simulink model "PMSM_DBPC"  (R2024b)
settings: Solver=FixedStepDiscrete  StartTime=0.0  StopTime=0.8  FixedStep=1e-6  RelTol=1e-3
libraries: spsMosfetLib x12, spsDiodeLib x6, spsCurrentMeasurementLib x6, spsVoltageMeasurementLib x5, spsSeriesRLCBranchLib x4, spsDCVoltageSourceLib x3, simulink x2, spsOnDelayLib x1, slpidlib x1, spsPermanentMagnetSynchronousMachineLib x1, spspowerguiLib x1
settings Model: Creator=23230  LastModifiedBy=23230

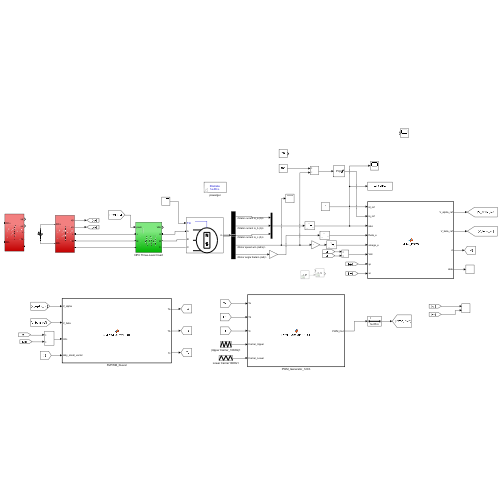
[thumbnail: Simulink's stored preview of the top-level diagram]
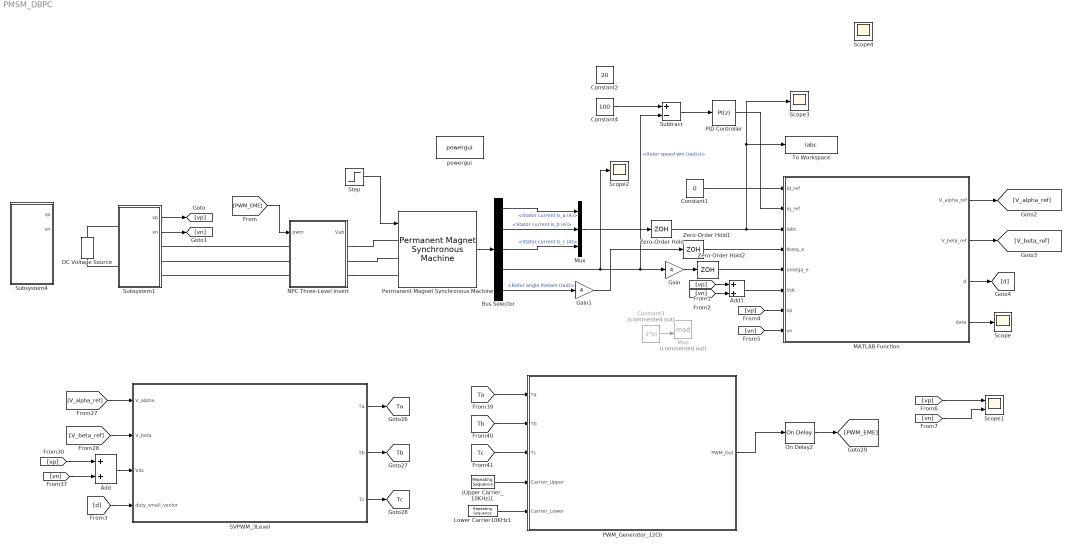
== system PMSM_DBPC ==
  (Upper Carrier_10KHz)1 : simulink/Sources/Repeating Sequence  rep_seq_t=[0, 5e-5, 1e-4]  rep_seq_y=[0.5, 1, 0.5]
  Add : Sum
  Add1 : Sum
  Bus Selector : BusSelector  OutputSignals=Stator current is_a (A),Stator current is_b (A),Stator current is_c (A),Rotor speed wm (rad/s),Rotor angle thetam (rad)
  Constant1 : Constant  Value=0
  Constant2 : Constant  Value=20
  Constant3 : Constant  Commented=on  Value=2*pi
  Constant4 : Constant  Value=100
  DC Voltage Source : spsDCVoltageSourceLib/DC Voltage Source  Amplitude=600  Measurements=None
  Gain : Gain  Gain=4
  Gain1 : Gain  Gain=4
  Lower Carrier10KHz1 : simulink/Sources/Repeating Sequence  rep_seq_t=[0, 5e-5, 1e-4]  rep_seq_y=[0, 0.5, 0]
  MATLAB Function : MATLAB Function  TreatAsAtomicUnit=on
  Mod : Math  Commented=on  Operator=mod
  Mux : Mux  Inputs=3
  NPC Three-Level Invert : Subsystem
  On Delay2 : spsOnDelayLib/On Delay  DelayType=On delay  delay=1e-6  ic=0  Ts=0
  PID Controller : slpidlib/PID Controller  Controller=PI  Form=Parallel  TimeDomain=Discrete-time  UseExternalTs=off  SampleTime=-1  IntegratorMethod=Forward Euler  FilterMethod=Forward Euler  ControllerParametersSource=internal  P=5  I=50  UseKiTs=off  D=0  UseExternalDerivativeSource=off  N=100  UseFilter=on  TunerSelectOption=Transfer Function Based (PID Tuner App)  InitialConditionSource=internal  InitialConditionForIntegrator=0  InitialConditionForFilter=0  DifferentiatorICPrevScaledInput=0  ExternalReset=none  TrackingMode=off  Kt=1  LimitOutput=on  SatLimitsSource=internal  UpperSaturationLimit=40  LowerSaturationLimit=-40  LinearizeAsGain=on  AntiWindupMode=none  Kb=1  LimitIntegrator=off  UpperIntegratorSaturationLimit=inf  LowerIntegratorSaturationLimit=-inf  POutMin=[]  POutMax=[]  IOutMin=[]  IOutMax=[]  DOutMin=[]  DOutMax=[]  NOutMin=[]  NOutMax=[]  SumOutMin=[]  SumOutMax=[]  SaturationOutMin=[]  SaturationOutMax=[]  PParamMin=[]  PParamMax=[]  IParamMin=[]  IParamMax=[]  DParamMin=[]  DParamMax=[]  NParamMin=[]  NParamMax=[]  KbParamMin=[]  KbParamMax=[]  KtParamMin=[]  KtParamMax=[]  KbOutMin=[]  KbOutMax=[]  KtOutMin=[]  KtOutMax=[]  IntegratorOutMin=[]  IntegratorOutMax=[]  FilterOutMin=[]  FilterOutMax=[]  SumI1OutMin=[]  SumI1OutMax=[]  SumI2OutMin=[]  SumI2OutMax=[]  SumI3OutMin=[]  SumI3OutMax=[]  SumI4OutMin=[]  SumI4OutMax=[]  SumDOutMin=[]  SumDOutMax=[]  DifferentiatorOutMin=[]  DifferentiatorOutMax=[]  FilterDiffOutCoefMin=[]  FilterDiffOutCoefMax=[]  ReciprocalOutMin=[]  ReciprocalOutMax=[]  SumDenOutMin=[]  SumDenOutMax=[]  SumNumOutMin=[]  SumNumOutMax=[]  DivideOutMin=[]  DivideOutMax=[]  UdiffTsProdOutMin=[]  UdiffTsProdOutMax=[]  NTsProdOutMin=[]  NTsProdOutMax=[]  UintegralTsProdOutMin=[]  UintegralTsProdOutMax=[]  UngainTsProdOutMin=[]  UngainTsProdOutMax=[]  ClampingZeroOutDataTypeStr=Inherit: Inherit via back propagation  ClampingZeroOutMin=[]  ClampingZeroOutMax=[]  FilterDenConstantOutDataTypeStr=Inherit: Inherit via back propagation  FilterDenConstantOutMin=[]  FilterDenConstantOutMax=[]  PCopyOutDataTypeStr=Inherit: Inherit via back propagation  PCopyOutMin=[]  PCopyOutMax=[]  NCopyOutDataTypeStr=Inherit: Inherit via back propagation  NCopyOutMin=[]  NCopyOutMax=[]  IntegratorContinuousStateAttributes=''  IntegratorStateMustResolveToSignalObject=off  IntegratorRTWStateStorageClass=Auto  FilterContinuousStateAttributes=''  FilterStateMustResolveToSignalObject=off  FilterRTWStateStorageClass=Auto  ParallelPVariant=InternalParameters  IdealPVariant=Disabled  IVariant=InternalParameters  DVariant=Disabled  IntegratorVariant=Discrete  SatVariant=Enabled  AWVariant=Passthrough  PCopyVariant=Disabled  TRVariant=Disabled  FdbkBlocksVariant=Forward  IdealPFdbkVariant=Disabled  SatFdbkVariant=Disabled  DerivativeFilterVariant=Disabled  NVariant=Disabled  NCopyVariant=Disabled_SignalSpec  FilterICVariant=Disabled  IntegratorICVariant=InternalICs  ExternalResetVariant=Disabled  TRSumVariant=Passthrough  SumFdbkVariant=Disabled  SumVariant=Sum_PI  TsampFilterVariant=InternalTs  TsampNgainVariant=Passthrough  TsampIntegralVariant=Disabled_SignalSpec  ExternalSaturationOutDataTypeStr=Inherit: Same as second input  DerivativeSourceVariant=Disabled  PreIntVariant=InternalPreInt
  PWM_Generator_12Ch : MATLAB Function  TreatAsAtomicUnit=on
  Permanent Magnet Synchronous Machine : spsPermanentMagnetSynchronousMachineLib/Permanent Magnet Synchronous Machine  NbPhases=3  FluxDistribution=Sinusoidal  RotorType=Round  MechanicalLoad=Torque Tm  PresetModel=No  ShowDetailedParameters=on  MeasurementBus=off  Resistance=0.015  Inductance=8.5e-3  dqInductances=[8.5e-3,8.5e-3]  La=0.00025  MachineConstant=Flux linkage established by magnets (V.s)  Flux=0.08  VoltageCst=58.0416  TorqueCst=0.48  Flat=120  Mechanical=[0.0027 0.0004924 4 0]  PolePairs=4  InitialConditions=[0,0, 0,0]  InitialConditions5ph=[0 0 0 0 0 0]  RefAngle=Aligned with phase A axis (original Park)  IterativeDiscreteModel=Trapezoidal non iterative  TsBlock=-1  TsPowergui=0
  SVPWM_3Level : MATLAB Function  TreatAsAtomicUnit=on
  Scope{,2..4} (4 alike) : Scope
  Scope1 : Scope  NumInputPorts=2
  Step : Step  Time=0.15  Before=5  After=15  SampleTime=0
  Subsystem1 : Subsystem
  Subsystem4 : Subsystem
  Subtract : Sum  Inputs=+-
  To Workspace : ToWorkspace  VariableName=iabc  SaveFormat=Timeseries  SampleTime=-1
  Zero-Order Hold : ZeroOrderHold  SampleTime=1e-4
  Zero-Order Hold1 : ZeroOrderHold  SampleTime=1e-4
  Zero-Order Hold2 : ZeroOrderHold  SampleTime=1e-4
  powergui : spspowerguiLib/powergui  Priority=1  SimulationMode=Discrete  SampleTime=1e-6  frequency=60  Iterations=50  frequencyindice=0  Pbase=100e6  ErrMax=1e-4  UnitsV=kV  UnitsW=MW  buscounter=0  FunctionMessages=off  echomessages=off  EnableUseOfTLC=off  CurrentSourceSwitches=off  DisableSnubberDevices=off  DisableRonSwitches=off  DisableVfSwitches=off  DisplayEquations=off  AutomaticDiscreteSolvers=off  SolverType=Tustin/Backward Euler (TBE)  Interpol=off  ExternalGateDelay=off  methode=off  Ts=100  x0status=blocks  SPID=on  SwTol=0  HookPort=off  NonlinearTolerance=1e-4  nMaxIteration=100  ContinueOnMaxIteration=off  RestoreLinks=warning  ResistiveCurrentMeasurement=off  Frange=[0:2:500]  Ylog=off  Xlog=on  ShowGrid=off  save=off  variable=ZData  structure=0  ZoomFFT=off  StartTime=0.0  cycles=1  DisplayStyle=1  fundamental=60  FreqAxis=off  MaxFrequency=1000  frequencyindicesteady=1  RmsSteady=1  display=off
  tag scope: Ta=global, Tb=global, Tc=global
  wires:
  Constant1/1 -> MATLAB Function/1(id_ref)
  [vp] -> Add/1
  [vn] -> Add/2
  [V_beta_ref] -> SVPWM_3Level/2(V_beta)
  [V_alpha_ref] -> SVPWM_3Level/1(V_alpha)
  SVPWM_3Level/1(Ta) -> [Ta]
  SVPWM_3Level/3(Tc) -> [Tc]
  SVPWM_3Level/2(Tb) -> [Tb]
  Add/1 -> SVPWM_3Level/3(Vdc)
  [Tc] -> PWM_Generator_12Ch/3(Tc)
  Lower Carrier10KHz1/1 -> PWM_Generator_12Ch/5(Carrier_Lower)
  On Delay2/1 -> [PWM_EME]
  (Upper Carrier_10KHz)1/1 -> PWM_Generator_12Ch/4(Carrier_Upper)
  PWM_Generator_12Ch/1(PWM_Out) -> On Delay2/1
  [Ta] -> PWM_Generator_12Ch/1(Ta)
  [Tb] -> PWM_Generator_12Ch/2(Tb)
  [PWM_EME] -> NPC Three-Level Invert/1(pwm)
  Permanent Magnet Synchronous Machine/1 -> Bus Selector/1
  Bus Selector/1 -> Mux/1  "<Stator current is_a (A)>"
  Bus Selector/2 -> Mux/2  "<Stator current is_b (A)>"
  Bus Selector/3 -> Mux/3  "<Stator current is_c (A)>"
  Mux/1 -> Zero-Order Hold/1
  Bus Selector/4 -> Scope2/1, Subtract/2, Gain/1  "<Rotor speed wm (rad/s)>"
  Gain/1 -> Zero-Order Hold2/1
  Bus Selector/5 -> Gain1/1  "<Rotor angle thetam (rad)>"
  Constant3/1 -> Mod/2
  [d] -> SVPWM_3Level/4(duty_small_vector)
  MATLAB Function/1(V_alpha_ref) -> [V_alpha_ref]
  MATLAB Function/2(V_beta_ref) -> [V_beta_ref]
  MATLAB Function/4(data) -> Scope/1
  [vn] -> Add1/2
  [vp] -> Add1/1
  Add1/1 -> MATLAB Function/6(Vdc)
  Zero-Order Hold/1 -> To Workspace/1, Scope3/1, MATLAB Function/3(iabc)
  Zero-Order Hold1/1 -> MATLAB Function/4(theta_e)
  Zero-Order Hold2/1 -> MATLAB Function/5(omega_e)
  Gain1/1 -> Zero-Order Hold1/1
  Subsystem1/1(vp) -> [vp]
  Subsystem1/2(vn) -> [vn]
  MATLAB Function/3(d) -> [d]
  [vp] -> MATLAB Function/7(vp)
  [vn] -> MATLAB Function/8(vn)
  [vp] -> Scope1/1
  [vn] -> Scope1/2
  Constant4/1 -> Subtract/1
  Subtract/1 -> PID Controller/1
  PID Controller/1 -> MATLAB Function/2(iq_ref)
  Step/1 -> Permanent Magnet Synchronous Machine/1
  connections:
  NPC Three-Level Invert/RConn1 -- Permanent Magnet Synchronous Machine/LConn1
  NPC Three-Level Invert/RConn2 -- Permanent Magnet Synchronous Machine/LConn2
  NPC Three-Level Invert/RConn3 -- Permanent Magnet Synchronous Machine/LConn3
  NPC Three-Level Invert/LConn1 -- Subsystem1/RConn1
  NPC Three-Level Invert/LConn2 -- Subsystem1/RConn2
  NPC Three-Level Invert/LConn3 -- Subsystem1/RConn3
  DC Voltage Source/RConn1 -- Subsystem1/LConn1
  DC Voltage Source/LConn1 -- Subsystem1/LConn2

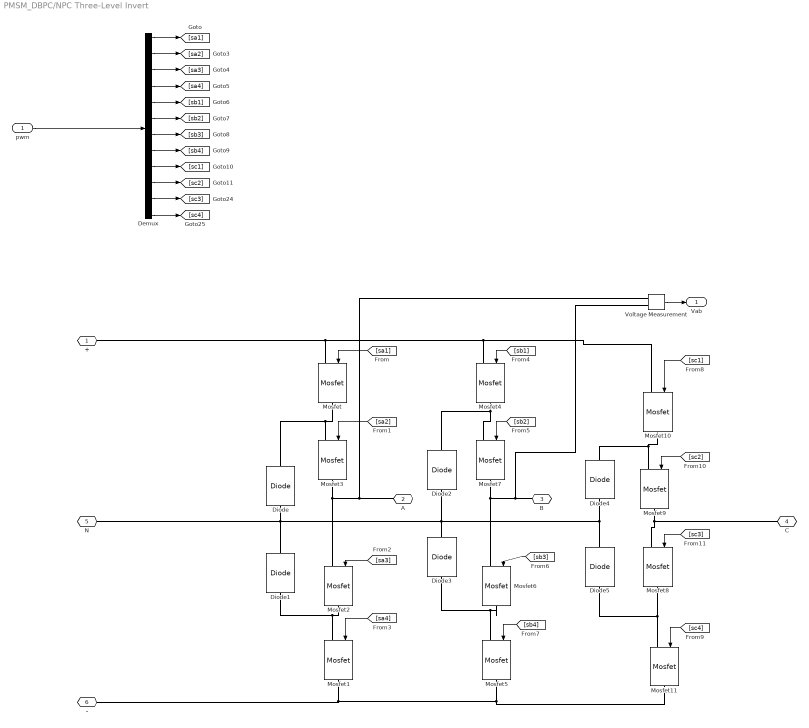
== system PMSM_DBPC/NPC Three-Level Invert ==
  pwm : Inport
  Demux : Demux  Outputs=12
  Diode{,1..5} (6 alike) : spsDiodeLib/Diode  Ron=0.001  Lon=0  Vf=0.8  IC=0  UseSnubber=0  Rs=500  Cs=250e-9  Measurements=off
  Mosfet{,1..11} (12 alike) : spsMosfetLib/Mosfet  Ron=0.1  Lon=0  Rd=0.01  Vfd=0  IC=0  Rs=1e5  Cs=inf  Measurements=off
  Voltage Measurement : spsVoltageMeasurementLib/Voltage Measurement  PhasorSimulation=off  OutputType=Complex  PSBequivalent=0
  + : PMIOPort  Side=Left
  A : PMIOPort  Port=2  Side=Right
  B : PMIOPort  Port=3  Side=Right
  C : PMIOPort  Port=4  Side=Right
  N : PMIOPort  Port=5  Side=Left
  - : PMIOPort  Port=6  Side=Left
  Vab : Outport
  wires:
  [sb2] -> Mosfet7/1
  [sc3] -> Mosfet8/1
  [sa4] -> Mosfet1/1
  Demux/2 -> [sa2]
  Demux/10 -> [sc2]
  Demux/7 -> [sb3]
  Demux/4 -> [sa4]
  Demux/11 -> [sc3]
  [sb3] -> Mosfet6/1
  [sc1] -> Mosfet10/1
  [sc4] -> Mosfet11/1
  Demux/9 -> [sc1]
  [sa1] -> Mosfet/1
  Demux/1 -> [sa1]
  Demux/12 -> [sc4]
  [sa3] -> Mosfet2/1
  [sc2] -> Mosfet9/1
  [sb1] -> Mosfet4/1
  Demux/5 -> [sb1]
  [sb4] -> Mosfet5/1
  [sa2] -> Mosfet3/1
  Demux/6 -> [sb2]
  Demux/3 -> [sa3]
  Demux/8 -> [sb4]
  Voltage Measurement/1 -> Vab/1
  pwm/1 -> Demux/1
  connections:
  Mosfet/RConn1 -- Diode/RConn1 -- Mosfet3/LConn1
  Mosfet9/RConn1 -- C/RConn1 -- Mosfet8/LConn1
  Mosfet9/LConn1 -- Diode4/RConn1 -- Mosfet10/RConn1
  Diode3/RConn1 -- Diode5/RConn1 -- Diode4/LConn1 -- Diode2/LConn1 -- Diode1/RConn1 -- N/RConn1 -- Diode/LConn1
  Mosfet/LConn1 -- +/RConn1 -- Mosfet10/LConn1 -- Mosfet4/LConn1
  Mosfet8/RConn1 -- Diode5/LConn1 -- Mosfet11/LConn1
  Mosfet2/RConn1 -- Diode1/LConn1 -- Mosfet1/LConn1
  Mosfet1/RConn1 -- -/RConn1 -- Mosfet11/RConn1 -- Mosfet5/RConn1
  Mosfet3/RConn1 -- Mosfet2/LConn1 -- Voltage Measurement/LConn1 -- A/RConn1
  Mosfet6/RConn1 -- Diode3/LConn1 -- Mosfet5/LConn1
  Mosfet7/RConn1 -- Mosfet6/LConn1 -- Voltage Measurement/LConn2 -- B/RConn1
  Mosfet4/RConn1 -- Diode2/RConn1 -- Mosfet7/LConn1

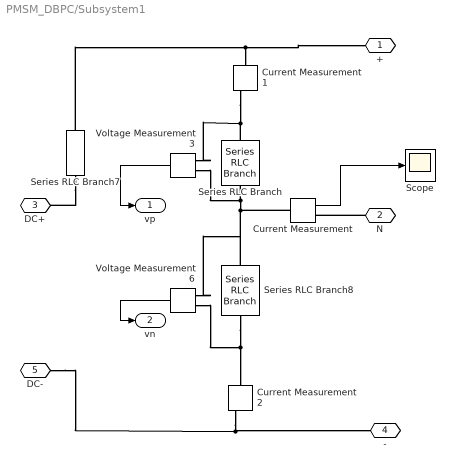
== system PMSM_DBPC/Subsystem1 ==
  Current Measurement : spsCurrentMeasurementLib/Current Measurement  PhasorSimulation=off  OutputType=Complex  PSBequivalent=0
  Current Measurement1 : spsCurrentMeasurementLib/Current Measurement  PhasorSimulation=off  OutputType=Complex  PSBequivalent=0
  Current Measurement2 : spsCurrentMeasurementLib/Current Measurement  PhasorSimulation=off  OutputType=Complex  PSBequivalent=0
  Scope : Scope
  Series RLC Branch : spsSeriesRLCBranchLib/Series RLC Branch  LConnTagsString=__new0  RConnTagsString=__new0  BranchType=C  Resistance=1  Inductance=1e-3  SetiL0=off  InitialCurrent=0  Capacitance=470e-6  Setx0=on  InitialVoltage=300  Measurements=Branch current
  Series RLC Branch7 : spsSeriesRLCBranchLib/Series RLC Branch  LConnTagsString=__new0  RConnTagsString=__new0  BranchType=R  Resistance=0.0001  Inductance=1e-3  SetiL0=off  InitialCurrent=0  Capacitance=1e-6  Setx0=off  InitialVoltage=0  Measurements=None
  Series RLC Branch8 : spsSeriesRLCBranchLib/Series RLC Branch  LConnTagsString=__new0  RConnTagsString=__new0  BranchType=C  Resistance=1  Inductance=1e-3  SetiL0=off  InitialCurrent=0  Capacitance=470e-6  Setx0=on  InitialVoltage=300  Measurements=Branch current
  Voltage Measurement3 : spsVoltageMeasurementLib/Voltage Measurement  PhasorSimulation=off  OutputType=Complex  PSBequivalent=0
  Voltage Measurement6 : spsVoltageMeasurementLib/Voltage Measurement  PhasorSimulation=off  OutputType=Complex  PSBequivalent=0
  + : PMIOPort  Side=Right
  N : PMIOPort  Port=2  Side=Right
  DC+ : PMIOPort  Port=3  Side=Left
  - : PMIOPort  Port=4  Side=Right
  DC- : PMIOPort  Port=5  Side=Left
  vp : Outport
  vn : Outport  Port=2
  wires:
  Voltage Measurement3/1 -> vp/1
  Voltage Measurement6/1 -> vn/1
  Current Measurement/1 -> Scope/1
  connections:
  Series RLC Branch7/RConn1 -- Current Measurement1/LConn1 -- +/RConn1
  Series RLC Branch/RConn1 -- Voltage Measurement3/LConn2 -- Series RLC Branch8/LConn1 -- Voltage Measurement6/LConn1 -- Current Measurement/LConn1
  Series RLC Branch8/RConn1 -- Current Measurement2/LConn1 -- Voltage Measurement6/LConn2
  Series RLC Branch7/LConn1 -- DC+/RConn1
  N/RConn1 -- Current Measurement/RConn1
  Current Measurement1/RConn1 -- Voltage Measurement3/LConn1 -- Series RLC Branch/LConn1
  Current Measurement2/RConn1 -- -/RConn1 -- DC-/RConn1

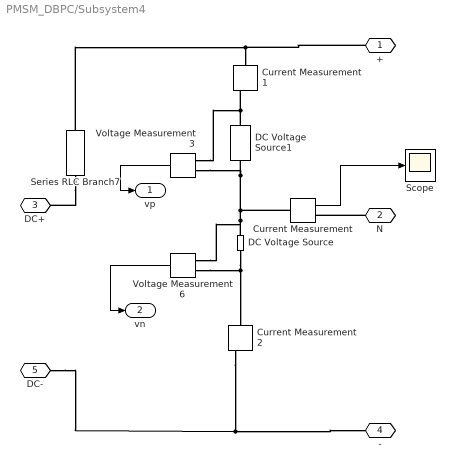
== system PMSM_DBPC/Subsystem4 ==
  Current Measurement : spsCurrentMeasurementLib/Current Measurement  PhasorSimulation=off  OutputType=Complex  PSBequivalent=0
  Current Measurement1 : spsCurrentMeasurementLib/Current Measurement  PhasorSimulation=off  OutputType=Complex  PSBequivalent=0
  Current Measurement2 : spsCurrentMeasurementLib/Current Measurement  PhasorSimulation=off  OutputType=Complex  PSBequivalent=0
  DC Voltage Source : spsDCVoltageSourceLib/DC Voltage Source  Amplitude=300  Measurements=None
  DC Voltage Source1 : spsDCVoltageSourceLib/DC Voltage Source  Amplitude=300  Measurements=None
  Scope : Scope
  Series RLC Branch7 : spsSeriesRLCBranchLib/Series RLC Branch  LConnTagsString=__new0  RConnTagsString=__new0  BranchType=R  Resistance=0.0001  Inductance=1e-3  SetiL0=off  InitialCurrent=0  Capacitance=1e-6  Setx0=off  InitialVoltage=0  Measurements=None
  Voltage Measurement3 : spsVoltageMeasurementLib/Voltage Measurement  PhasorSimulation=off  OutputType=Complex  PSBequivalent=0
  Voltage Measurement6 : spsVoltageMeasurementLib/Voltage Measurement  PhasorSimulation=off  OutputType=Complex  PSBequivalent=0
  + : PMIOPort  Side=Right
  N : PMIOPort  Port=2  Side=Right
  DC+ : PMIOPort  Port=3  Side=Left
  - : PMIOPort  Port=4  Side=Right
  DC- : PMIOPort  Port=5  Side=Left
  vp : Outport
  vn : Outport  Port=2
  wires:
  Voltage Measurement3/1 -> vp/1
  Voltage Measurement6/1 -> vn/1
  Current Measurement/1 -> Scope/1
  connections:
  Series RLC Branch7/RConn1 -- +/RConn1 -- Current Measurement1/LConn1
  DC Voltage Source/LConn1 -- Current Measurement2/LConn1 -- Voltage Measurement6/LConn2
  Series RLC Branch7/LConn1 -- DC+/RConn1
  N/RConn1 -- Current Measurement/RConn1
  Current Measurement2/RConn1 -- -/RConn1 -- DC-/RConn1
  DC Voltage Source1/RConn1 -- Voltage Measurement3/LConn1 -- Current Measurement1/RConn1
  DC Voltage Source/RConn1 -- Voltage Measurement3/LConn2 -- DC Voltage Source1/LConn1 -- Current Measurement/LConn1 -- Voltage Measurement6/LConn1

== matlab function PMSM_DBPC/MATLAB Function ==
  data: id_ref input; V_alpha_ref output; iq_ref input; iabc input; theta_e input; omega_e input; Vdc input; V_beta_ref output; d output; data output; vp input; vn input
function [V_alpha_ref, V_beta_ref, d, data] = Motor_DBPC(id_ref, iq_ref, iabc, theta_e, omega_e, Vdc, vp, vn)
    % ==========================================================
    % 永磁同步电机多目标解析无差拍预测控制 (MO-DBPC) 
    % 包含：1. 前馈+抗饱和条件积分复合控制 (彻底消除稳态静差且防爆炸)
    %       2. 基于电荷预测的多目标中点电位平衡控制
    % ==========================================================
    
    % --- 0. 物理参数定义 ---
    Ts = 1e-4;         % 采样周期 (s)
    Rs = 0.015;        % 定子电阻 (Ohm)
    Ld = 0.00025;      % d轴电感 (H)
    Lq = 0.00025;      % q轴电感 (H)
    psi_f = 0.08;      % 永磁体磁链 (Wb)
    C_cap = 470e-6;    % 直流侧单电容容量 (F)
    
    % --- 1. 坐标变换 (abc -> alpha/beta -> d/q) ---
    T_clark = (2/3) * [1, -0.5, -0.5; 0, sqrt(3)/2, -sqrt(3)/2];
    i_ab = T_clark * iabc;
    i_alpha = i_ab(1);
    i_beta  = i_ab(2);
    
    id =  i_alpha * cos(theta_e) + i_beta * sin(theta_e);
    iq = -i_alpha * sin(theta_e) + i_beta * cos(theta_e);
    
    % --- 2. 电流追踪：前馈无差拍 + 条件积分补偿 (消除静差) ---
    % 声明持久化变量，作为离散积分器的记忆单元
    persistent ud_int uq_int;
    if isempty(ud_int)
        ud_int = 0;
        uq_int = 0;
    end
    
    % 积分控制器参数 (针对 1e-4 极小步长优化)
    Ki = 0.005;        % 极小积分增益，保证稳态微调的平滑性
    Int_Limit = 15;    % 积分抗饱和限幅值 (V)，防止超调翻车
    
    % 计算当前拍的电流静差
    err_d = id_ref - id;
    err_q = iq_ref - iq;
    
    % 【核心修复】：条件积分 (Conditional Integration)
    % 仅在误差小于 5A 时开启积分，完美避开启动和突加负载瞬间的 Windup 爆炸
    if abs(err_d) < 5
        ud_int = ud_int + Ki * err_d;
    end
    
    if abs(err_q) < 5
        uq_int = uq_int + Ki * err_q;
    end
    
    % 抗饱和限幅 (最后的一道安全锁)
    ud_int = max(-Int_Limit, min(Int_Limit, ud_int));
    uq_int = max(-Int_Limit, min(Int_Limit, uq_int));
    
    % 复合控制电压求解：DBPC物理前馈(定大局) + 误差积分补偿(修毫厘)
    ud_ref = Rs * id + (Ld / Ts) * (id_ref - id) - omega_e * Lq * iq + ud_int;
    uq_ref = Rs * iq + (Lq / Ts) * (iq_ref - iq) + omega_e * Ld * id + omega_e * psi_f + uq_int;
    
    % --- 3. 逆坐标变换 (d/q -> alpha/beta) ---
    V_alpha_ref = ud_ref * cos(theta_e) - uq_ref * sin(theta_e);
    V_beta_ref  = ud_ref * sin(theta_e) + uq_ref * cos(theta_e);
    
    % --- 4. 【核心创新】：改进多目标解析无差拍中点控制 ---
    delta_v = vp - vn; % 当前中点电压偏差
    
    % 扇区判断 (根据参考电压矢量定位)
    theta_v = atan2(V_beta_ref, V_alpha_ref);
    if theta_v < 0, theta_v = theta_v + 2*pi; end
    Sector = floor(theta_v / (pi/3)) + 1;
    if Sector > 6, Sector = 6; end
    
    % 根据扇区提取可能流过中点的相电流
    switch Sector
        case 1, i_p = iabc(1);  i_n = -iabc(1); 
        case 2, i_p = -iabc(3); i_n = iabc(3);
        case 3, i_p = iabc(2);  i_n = -iabc(2);
        case 4, i_p = -iabc(1); i_n = iabc(1);
        case 5, i_p = iabc(3);  i_n = -iabc(3);
        case 6, i_p = -iabc(2); i_n = iabc(2);
        otherwise, i_p = 0; i_n = 0;
    end
    
    % 解析求解最优分配因子 d
    denominator = i_p - i_n;
    if abs(denominator) < 0.1
        % 如果中点电流激励过小，为防止除以0的奇异点，直接均分
        d = 0.5; 
    else
        % 多目标解析解：兼顾电压平衡 (lambda_v) 与 电流平滑 (lambda_cmv)
        lambda_v   = 1.0;  
        lambda_cmv = 0.005; % THD与电压波动的最优折中权重
        
        % 代价函数求导后的代数解析解计算
        A = (Ts / C_cap) * denominator;
        V_req = delta_v - (Ts / C_cap) * i_n;
        d = (lambda_v * A * V_req + 0.5 * lambda_cmv) / (lambda_v * A^2 + lambda_cmv);
    end
    
    % 占空比物理约束
    d = max(0.0, min(1.0, d));
    
    % 导出数据供示波器观察
    data = [id; iq; id_ref; iq_ref; delta_v; d]; 
end

== matlab function PMSM_DBPC/SVPWM_3Level ==
  data: V_alpha input; Ta output; V_beta input; Vdc input; duty_small_vector input; Tb output; Tc output
function [Ta, Tb, Tc] = SVPWM_3Level_Full(V_alpha, V_beta, Vdc, duty_small_vector)
    % ==========================================================
    % 三电平 NPC 逆变器空间矢量调制 (全扇区映射版)
    % 集成 DBPC 冗余小矢量非对称分配 (协同控制电容电压与零序电流)
    % 【最终完美版】：已修复 atan2 下半圆负角度导致的停工 Bug
    % ==========================================================
    
    % --- 1. 参考电压极坐标转换 ---
    V_ref = sqrt(V_alpha^2 + V_beta^2);
    theta = atan2(V_beta, V_alpha);
    
    % ==========================================================
    % 【救命补丁：防止下半平面角度变负数，导致逆变器罢工！】
    % ==========================================================
    if theta < 0
        theta = theta + 2*pi;
    end
    
    % 计算调制比
    m = sqrt(3) * V_ref / Vdc; 
    
    % --- 2. 扇区判断 (Sector 1 ~ 6) ---
    Sector = floor(theta / (pi/3)) + 1;
    if Sector > 6
        Sector = 6; % 安全保护
    end
    
    % --- 3. 核心：扇区对称映射 ---
    if mod(Sector, 2) == 0
        theta_rel = pi/3 - mod(theta, pi/3);
    else
        theta_rel = mod(theta, pi/3);
    end
    
    % --- 4. 计算基础变量 X, Y, Z ---
    X = m * sin(pi/3 - theta_rel);
    Y = m * sin(theta_rel);
    Z = X + Y;
    
    % 提取协同控制因数 d
    d = duty_small_vector;
    
    % --- 5. 区域判断与映射占空比计算 (D1, D2, D3) ---
    if Z <= 0.5
        D1 = 0.5 + Z * d;
        D2 = 0.5 - X + Z * d;
        D3 = 0.5 - Z * (1 - d);
    elseif X > 0.5
        D1 = 1 - (1 - Z) * (1 - d);
        D2 = Y + (1 - Z) * d;
        D3 = (1 - Z) * d;
    elseif Y > 0.5
        D1 = Y + (1 - Z) * d;
        D2 = 1 - (1 - Z) * (1 - d);
        D3 = (1 - Z) * d;
    else
        D1 = Z + (1 - Z) * d;
        D2 = Y + (1 - Z) * d;
        D3 = (1 - Z) * d;
    end
    
    % --- 6. 逆映射：分配给三相桥臂 (Ta, Tb, Tc) ---
    switch Sector
        case 1
            Ta = D1; Tb = D2; Tc = D3;
        case 2
            Ta = D2; Tb = D1; Tc = D3;
        case 3
            Ta = D3; Tb = D1; Tc = D2;
        case 4
            Ta = D3; Tb = D2; Tc = D1;
        case 5
            Ta = D2; Tb = D3; Tc = D1;
        case 6
            Ta = D1; Tb = D3; Tc = D2;
        otherwise
            Ta = 0.5; Tb = 0.5; Tc = 0.5;
    end
    
    % --- 7. 占空比硬限幅保护 ---
    Ta = max(0, min(1, Ta));
    Tb = max(0, min(1, Tb));
    Tc = max(0, min(1, Tc));
end

== matlab function PMSM_DBPC/PWM_Generator_12Ch ==
  data: Ta input; PWM_Out output; Tb input; Tc input; Carrier_Upper input; Carrier_Lower input
function PWM_Out = PWM_Generator_12Ch(Ta, Tb, Tc, Carrier_Upper, Carrier_Lower)
    % 三电平 12路 PWM 脉冲生成器
    % 输入:
    % Ta, Tb, Tc: 三相占空比 (0~1)
    % Carrier_Upper: 上层高频三角载波 (0.5~1)
    % Carrier_Lower: 下层高频三角载波 (0~0.5)
    
    % --- A相逻辑 ---
    sa1 = Ta >= Carrier_Upper;
    sa2 = Ta >= Carrier_Lower;
    sa3 = ~sa1; % 互补逻辑
    sa4 = ~sa2;

    % --- B相逻辑 ---
    sb1 = Tb >= Carrier_Upper;
    sb2 = Tb >= Carrier_Lower;
    sb3 = ~sb1;
    sb4 = ~sb2;

    % --- C相逻辑 ---
    sc1 = Tc >= Carrier_Upper;
    sc2 = Tc >= Carrier_Lower;
    sc3 = ~sc1;
    sc4 = ~sc2;

    % --- 打包输出 ---
    % 严格对应物理拓扑解复用器 (Demux) 的 12 路顺序打包为列向量
    PWM_Out = double([sa1; sa2; sa3; sa4; sb1; sb2; sb3; sb4; sc1; sc2; sc3; sc4]);
end
